simulink model "EEG_2022_040_Simulink_ex1"  (R2024a)
settings: Solver=VariableStepAuto  StartTime=0.0  StopTime=40  RelTol=1e-3
settings Model: Creator=User  LastModifiedBy=User

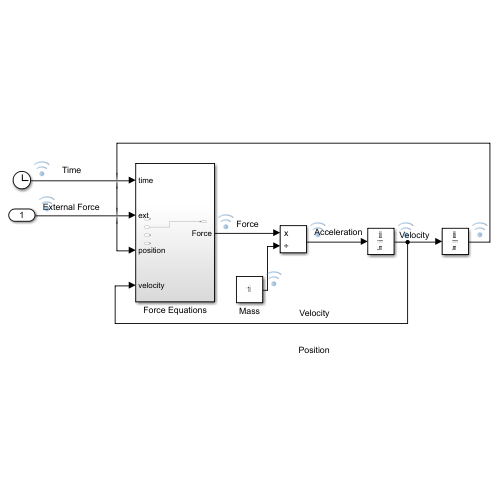
[thumbnail: Simulink's stored preview of the top-level diagram]
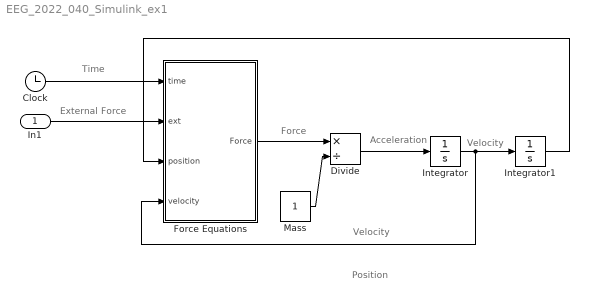
== system EEG_2022_040_Simulink_ex1 ==
  note: Velocity
  note: Time
  note: External Force
  note: Position
  note: Force
  note: Acceleration
  note: Velocity
  In1 : Inport
  Clock : Clock
  Divide : Product  Inputs=*/
  Force Equations : Subsystem
  Integrator : Integrator
  Integrator1 : Integrator
  Mass : Constant
  wires:
  Clock/1 -> Force Equations/1(time)
  In1/1 -> Force Equations/2(ext)
  Divide/1 -> Integrator/1
  Force Equations/1(Force) -> Divide/1
  Integrator/1 -> Integrator1/1, Force Equations/4(velocity)
  Integrator1/1 -> Force Equations/3(position)
  Mass/1 -> Divide/2

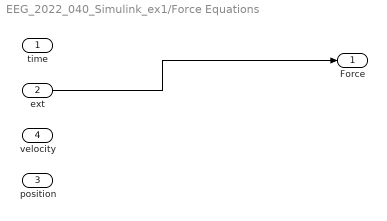
== system EEG_2022_040_Simulink_ex1/Force Equations ==
  time : Inport
  ext : Inport  Port=2
  position : Inport  Port=3
  velocity : Inport  Port=4
  Force : Outport
  wires:
  ext/1 -> Force/1
